simulink model "SVPWMv1"  (R2013a)
settings: Solver=ode45  StartTime=0.0  StopTime=2  MaxStep=.0001  RelTol=1e-3
libraries: powerlib x15, simulink x3, powerlib_meascontrol x1
settings Model: Creator=TELE  LastModifiedBy=TELE

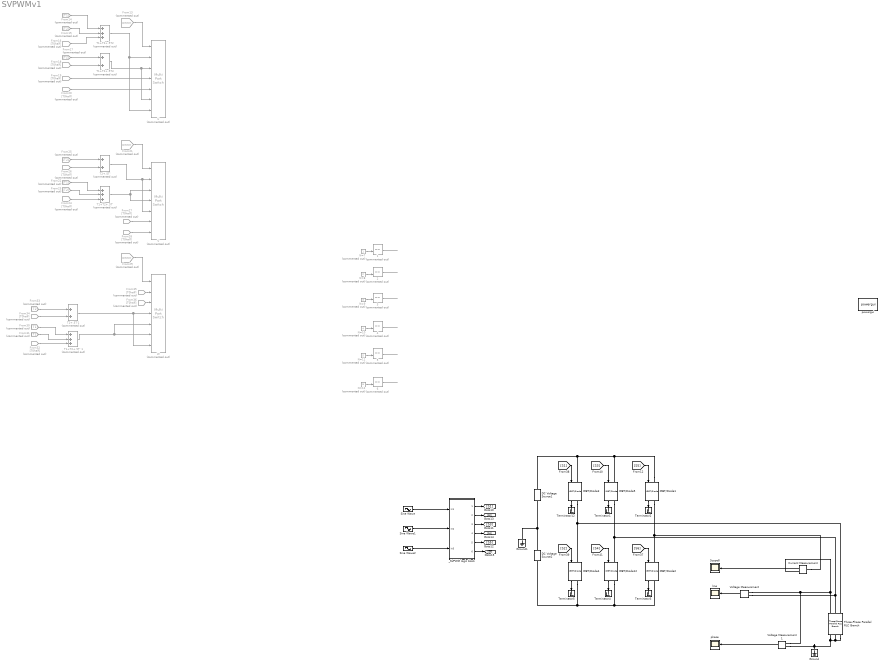
== system SVPWMv1 ==
  {1..6} (6 alike) : RelationalOperator  Commented=on  Operator===  OutDataTypeStr=boolean
  Current Measurement : powerlib/Measurements/Current Measurement  PhasorSimulation=off  OutputType=Complex  PSBequivalent=0
  DC Voltage Source1 : powerlib/Electrical Sources/DC Voltage Source  Amplitude=150  Measurements=None
  DC Voltage Source2 : powerlib/Electrical Sources/DC Voltage Source  Amplitude=150  Measurements=None
  From13 : From  Commented=on  GotoTag=sector
  From14 : From  Commented=on  GotoTag=T1
  From{15,17,23,25,31,33} (6 alike) : From  Commented=on  GotoTag=T2
  From{16,18..20,24,26..28,32,34..36} (12 alike) : From  Commented=on  GotoTag=T0half
  From21 : From  Commented=on  GotoTag=sector
  From22 : From  Commented=on  GotoTag=T1
  From29 : From  Commented=on  GotoTag=sector
  From30 : From  Commented=on  GotoTag=T1
  Ground : powerlib/Elements/Ground  LConnTagsString=a
  Ground1 : powerlib/Elements/Ground  LConnTagsString=a
  IGBT/Diode{1..5,12} (6 alike) : powerlib/Power Electronics/IGBT//Diode  Ron=1e-3  Rs=1e5  Cs=inf  Measurements=on
  N=10 : Constant  Commented=on  Value=4
  N=11 : Constant  Commented=on  Value=5
  N=12 : Constant  Commented=on  Value=6
  N=7 : Constant  Commented=on
  N=8 : Constant  Commented=on  Value=2
  N=9 : Constant  Commented=on  Value=3
  Scope8 : Scope
      settings: YMin=-600000  YMax=350000  SaveName=current
  Sine Wave : Sin  Frequency=50*2*pi  SampleTime=0
  Sine Wave1 : Sin  Frequency=50*2*pi  Phase=pi*(-2/3)  SampleTime=0
  Sine Wave2 : Sin  Frequency=50*2*pi  Phase=pi*(2/3)  SampleTime=0
  "T1+T2+.5T' " : Sum  Commented=on  Inputs=+++
  T1+T2+.5T' 1 : Sum  Commented=on  Inputs=+++
  T1+T2+.5T2 : Sum  Commented=on  Inputs=+++
  T1+T2+.5T3 : Sum  Commented=on  Inputs=2
  T2+.5T' : Sum  Commented=on  Inputs=2
  T2+.5T'1 : Sum  Commented=on  Inputs=2
  Terminator{1..5,12} (6 alike) : Terminator
  Three-Phase Parallel RLC Branch : powerlib/Elements/Three-Phase Parallel RLC Branch  LConnTagsString=A|B|C  RConnTagsString=A|B|C  BranchType=RLC  Resistance=100  Inductance=100e-3  Capacitance=100e-3  Measurements=None
  U : MultiPortSwitch  Commented=on  DataPortOrder=Specify indices  Inputs=4  DataPortIndices={1,2,3,4,5,6}
  V : MultiPortSwitch  Commented=on  DataPortOrder=Specify indices  Inputs=4  DataPortIndices={1,2,3,4,5,6}
  Voltage Measurement : powerlib/Measurements/Voltage Measurement  PhasorSimulation=off  OutputType=Complex  PSBequivalent=0
  Voltage Measurement1 : powerlib/Measurements/Voltage Measurement  PhasorSimulation=off  OutputType=Complex  PSBequivalent=0
  W : MultiPortSwitch  Commented=on  DataPortOrder=Specify indices  Inputs=4  DataPortIndices={1,2,3,4,5,6}
  _SVPWM logic block : Subsystem
  line : Scope
      settings: TimeRange=2  YMin=-175  YMax=175  SaveName=voltage
  phase : Scope
      settings: YMin=-10  YMax=150  SaveName=voltage1
  powergui : powerlib/powergui  Priority=1  SimulationMode=Continuous  SolverType=Tustin  SampleTime=50e-6  frequency=60  SPID=off  DisableSnubberDevices=off  DisableRonSwitches=off  DisableVfSwitches=off  SwTol=0  Interpol=off  DisplayEquations=off  frequencyindice=0  Pbase=100e6  ErrMax=1e-4  Iterations=50  UnitsV=kV  UnitsW=MW  FunctionMessages=off  echomessages=off  HookPort=off  EnableUseOfTLC=off  x0status=blocks  RestoreLinks=warning  ResistiveCurrentMeasurement=off  Frange=[0:2:500]  Ylog=off  Xlog=on  ShowGrid=off  save=off  variable=ZData  structure=voltage  ZoomFFT=off  StartTime=0.0  cycles=50  DisplayStyle=1  fundamental=50  FreqAxis=off  MaxFrequency=1000  frequencyindicesteady=1  RmsSteady=1  display=off  Ts=0  methode=off
  wires:
  ? -> 6/1, 5/1, 4/1, 3/1, 2/1, 1/1
  N=7/1 -> 1/2
  N=8/1 -> 2/2
  N=9/1 -> 3/2
  N=10/1 -> 4/2
  N=11/1 -> 5/2
  N=12/1 -> 6/2
  1/1 -> ?
  2/1 -> ?
  3/1 -> ?
  4/1 -> ?
  5/1 -> ?
  6/1 -> ?
  From13/1 -> U/1
  T1+T2+.5T2/1 -> U/2, U/7
  From14/1 -> T1+T2+.5T2/1
  From15/1 -> T1+T2+.5T2/2
  From16/1 -> T1+T2+.5T2/3
  From17/1 -> T1+T2+.5T3/1
  From18/1 -> T1+T2+.5T3/2
  T1+T2+.5T3/1 -> U/3, U/6
  From19/1 -> U/4
  From20/1 -> U/5
  From21/1 -> V/1
  From22/1 -> "T1+T2+.5T' "/1
  From23/1 -> "T1+T2+.5T' "/2
  From24/1 -> "T1+T2+.5T' "/3
  From25/1 -> T2+.5T'/1
  From26/1 -> T2+.5T'/2
  "T1+T2+.5T' "/1 -> V/4, V/3
  T2+.5T'/1 -> V/5, V/2
  From27/1 -> V/6
  From28/1 -> V/7
  From29/1 -> W/1
  From30/1 -> T1+T2+.5T' 1/1
  From31/1 -> T1+T2+.5T' 1/2
  From32/1 -> T1+T2+.5T' 1/3
  From33/1 -> T2+.5T'1/1
  From34/1 -> T2+.5T'1/2
  From35/1 -> W/2
  From36/1 -> W/3
  T2+.5T'1/1 -> W/7, W/4
  T1+T2+.5T' 1/1 -> W/6, W/5
  Voltage Measurement/1 -> line/1
  Current Measurement/1 -> Scope8/1
  Voltage Measurement1/1 -> phase/1
  _SVPWM logic block/6(6) -> [S6]
  [S6] -> IGBT/Diode2/1
  IGBT/Diode1/1 -> Terminator2/1
  _SVPWM logic block/2(2) -> [S2]
  IGBT/Diode4/1 -> Terminator5/1
  [S1] -> IGBT/Diode3/1
  IGBT/Diode5/1 -> Terminator1/1
  Sine Wave/1 -> _SVPWM logic block/1(In1)
  _SVPWM logic block/4(4) -> [S4]
  _SVPWM logic block/1(1) -> [S1]
  IGBT/Diode3/1 -> Terminator12/1
  IGBT/Diode2/1 -> Terminator3/1
  Sine Wave2/1 -> _SVPWM logic block/3(In3)
  [S3] -> IGBT/Diode5/1
  _SVPWM logic block/3(3) -> [S3]
  [S2] -> IGBT/Diode4/1
  [S5] -> IGBT/Diode1/1
  IGBT/Diode12/1 -> Terminator4/1
  [S4] -> IGBT/Diode12/1
  _SVPWM logic block/5(5) -> [S5]
  Sine Wave1/1 -> _SVPWM logic block/2(In2)
  connections:
  Voltage Measurement1/LConn2 -- Ground/LConn1 -- Three-Phase Parallel RLC Branch/LConn1 -- Three-Phase Parallel RLC Branch/LConn3 -- Three-Phase Parallel RLC Branch/LConn2
  DC Voltage Source1/LConn1 -- Ground1/LConn1 -- DC Voltage Source2/RConn1
  IGBT/Diode1/LConn1 -- DC Voltage Source1/RConn1 -- IGBT/Diode3/LConn1 -- IGBT/Diode5/LConn1
  IGBT/Diode2/RConn1 -- IGBT/Diode12/RConn1 -- DC Voltage Source2/LConn1 -- IGBT/Diode4/RConn1
  Voltage Measurement/LConn1 -- Current Measurement/RConn1 -- Three-Phase Parallel RLC Branch/RConn1 -- Voltage Measurement1/LConn1
  Voltage Measurement/LConn2 -- IGBT/Diode12/LConn1 -- IGBT/Diode5/RConn1 -- Three-Phase Parallel RLC Branch/RConn2
  IGBT/Diode3/RConn1 -- Three-Phase Parallel RLC Branch/RConn3 -- IGBT/Diode4/LConn1
  IGBT/Diode1/RConn1 -- Current Measurement/LConn1 -- IGBT/Diode2/LConn1

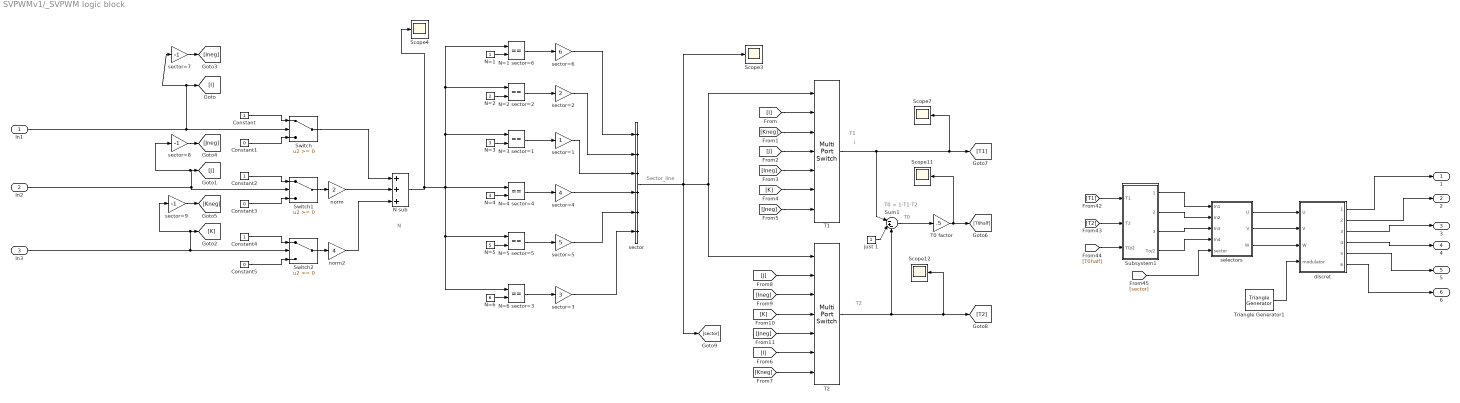
== system SVPWMv1/_SVPWM logic block ==
  note: T0
  note: T0 = 1-T1-T2
  note: T2
  note: T1
  note: i
  note: Sector_line
  note: N
  In1 : Inport
  In2 : Inport  Port=2
  In3 : Inport  Port=3
  Constant : Constant
  Constant1 : Constant  Value=0
  Constant2 : Constant
  Constant3 : Constant  Value=0
  Constant4 : Constant
  Constant5 : Constant  Value=0
  N sub : Sum  Inputs=+++
  N=1 : Constant
  N=1 sector=6 : RelationalOperator  Operator===  OutDataTypeStr=boolean
  N=2 : Constant  Value=2
  N=2 sector=2 : RelationalOperator  Operator===  OutDataTypeStr=boolean
  N=3 : Constant  Value=3
  N=3 sector=1 : RelationalOperator  Operator===  OutDataTypeStr=boolean
  N=4 : Constant  Value=4
  N=4 sector=4 : RelationalOperator  Operator===  OutDataTypeStr=boolean
  N=5 : Constant  Value=5
  N=5 sector=5 : RelationalOperator  Operator===  OutDataTypeStr=boolean
  N=6 : Constant  Value=6
  N=6 sector=3 : RelationalOperator  Operator===  OutDataTypeStr=boolean
  Scope{3..4,7,11..12} (5 alike) : Scope
      Scope11 settings: YMin=2.77556e-17  YMax=0.9  SaveName=current2
      Scope12 settings: YMin=2.77556e-17  YMax=0.9  SaveName=current3
      Scope3 settings: SaveName=ScopeData3
      Scope4 settings: SaveName=ScopeData4
      Scope7 settings: YMin=2.77556e-17  YMax=0.9  SaveName=current1
  Subsystem1 : Subsystem
  Sum1 : Sum  Inputs=|-+-
  Switch : Switch
  Switch1 : Switch
  Switch2 : Switch
  T0 factor : Gain  Gain=.5
  T1 : MultiPortSwitch  DataPortOrder=Specify indices  Inputs=4  DataPortIndices={1,2,3,4,5,6}
  T2 : MultiPortSwitch  DataPortOrder=Specify indices  Inputs=4  DataPortIndices={1,2,3,4,5,6}
  Triangle Generator1 : powerlib_meascontrol/Pulse & Signal Generators/Triangle Generator  Freq=50e3  Phase=180  Ts=0
  discret : Subsystem
  just 1 : Constant
  norm : Gain  Gain=2
  norm2 : Gain  Gain=4
  sector : Sum  Inputs=++++++
  sector=1 : Gain
  sector=2 : Gain  Gain=2
  sector=3 : Gain  Gain=3
  sector=4 : Gain  Gain=4
  sector=5 : Gain  Gain=5
  sector=6 : Gain  Gain=6
  sector=7 : Gain  Gain=-1
  sector=8 : Gain  Gain=-1
  sector=9 : Gain  Gain=-1
  selectors : Subsystem
  1 : Outport
  2 : Outport  Port=2
  3 : Outport  Port=3
  4 : Outport  Port=4
  5 : Outport  Port=5
  6 : Outport  Port=6
  wires:
  Constant1/1 -> Switch/3
  In1/1 -> Switch/2, sector=7/1, [I]
  Constant2/1 -> Switch1/1
  Constant/1 -> Switch/1
  Constant3/1 -> Switch1/3
  N=1/1 -> N=1 sector=6/2
  N=6/1 -> N=6 sector=3/2
  N=6 sector=3/1 -> sector=3/1
  N=5/1 -> N=5 sector=5/2
  N sub/1 -> Scope4/1, N=6 sector=3/1, N=5 sector=5/1, N=4 sector=4/1, N=3 sector=1/1, N=2 sector=2/1, N=1 sector=6/1
  N=3 sector=1/1 -> sector=1/1
  N=3/1 -> N=3 sector=1/2
  Constant4/1 -> Switch2/1
  Switch/1 -> N sub/1
  In2/1 -> Switch1/2, [J], sector=8/1
  N=4/1 -> N=4 sector=4/2
  N=5 sector=5/1 -> sector=5/1
  Switch2/1 -> norm2/1
  N=2/1 -> N=2 sector=2/2
  sector=2/1 -> sector/2
  N=2 sector=2/1 -> sector=2/1
  sector=4/1 -> sector/4
  sector=5/1 -> sector/5
  N=4 sector=4/1 -> sector=4/1
  sector=1/1 -> sector/3
  Switch1/1 -> norm/1
  sector=3/1 -> sector/6
  N=1 sector=6/1 -> sector=6/1
  sector=6/1 -> sector/1
  In3/1 -> Switch2/2, sector=9/1, [K]
  Constant5/1 -> Switch2/3
  [I] -> T1/2
  [Kneg] -> T2/7
  sector=8/1 -> [Jneg]
  Sum1/1 -> T0 factor/1
  T0 factor/1 -> Scope11/1, [T0half]
  sector/1 -> [sector], Scope3/1, T2/1, T1/1
  [Ineg] -> T1/5
  sector=7/1 -> [Ineg]
  norm2/1 -> N sub/3
  [Jneg] -> T1/7
  [J] -> T2/2
  [K] -> T1/6
  [J] -> T1/4
  [I] -> T2/6
  [K] -> T2/4
  T1/1 -> Scope7/1, [T1], Sum1/1
  sector=9/1 -> [Kneg]
  just 1/1 -> Sum1/2
  [Kneg] -> T1/3
  [Jneg] -> T2/5
  norm/1 -> N sub/2
  [Ineg] -> T2/3
  selectors/3(W) -> discret/3(W)
  Triangle Generator1/1 -> discret/4(modulator)
  discret/2(2) -> 2/1
  discret/3(3) -> 3/1
  Subsystem1/2(T1+To/2) -> selectors/2(In2)
  discret/4(4) -> 4/1
  Subsystem1/1(T1+T2+To/2) -> selectors/1(In1)
  [T1] -> Subsystem1/1(T1)
  [T0half] -> Subsystem1/3(T0/2)
  discret/1(1) -> 1/1
  T2/1 -> Sum1/3, Scope12/1, [T2]
  [T2] -> Subsystem1/2(T2)
  selectors/2(V) -> discret/2(V)
  Subsystem1/4(To/2) -> selectors/4(In4)
  [sector] -> selectors/5("sector ")
  Subsystem1/3(T2+To/2) -> selectors/3(In3)
  selectors/1(U) -> discret/1(U)
  discret/5(5) -> 5/1
  discret/6(6) -> 6/1

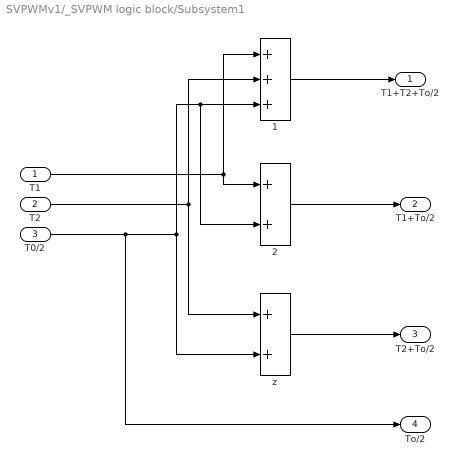
== system SVPWMv1/_SVPWM logic block/Subsystem1 ==
  T1 : Inport
  T2 : Inport  Port=2
  T0/2 : Inport  Port=3
  1 : Sum  Inputs=+++
  2 : Sum
  z : Sum
  T1+T2+To/2 : Outport
  T1+To/2 : Outport  Port=2
  T2+To/2 : Outport  Port=3
  To/2 : Outport  Port=4
  wires:
  T1/1 -> 2/1, 1/1
  T0/2/1 -> z/2, 1/3, 2/2, To/2/1
  2/1 -> T1+To/2/1
  1/1 -> T1+T2+To/2/1
  T2/1 -> z/1, 1/2
  z/1 -> T2+To/2/1

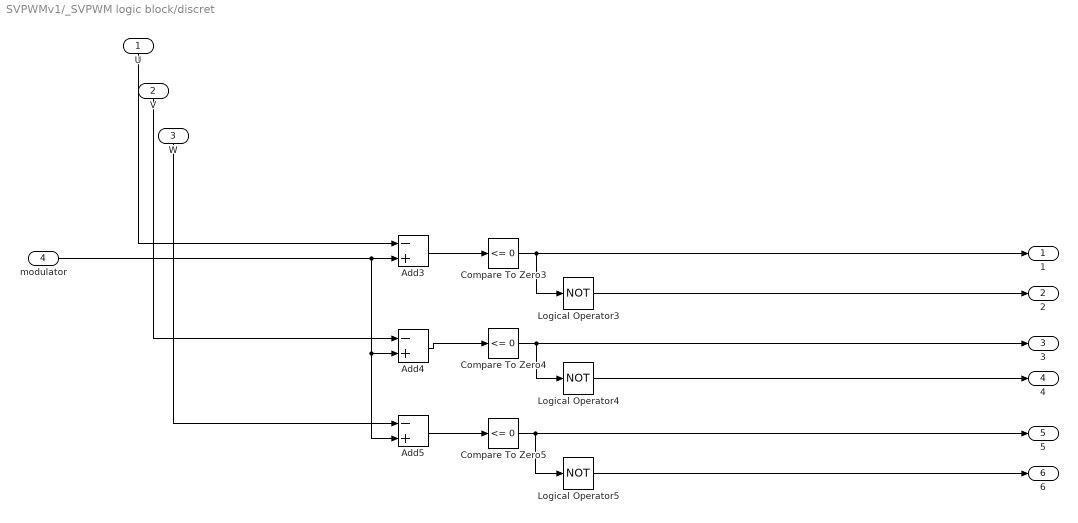
== system SVPWMv1/_SVPWM logic block/discret ==
  U : Inport
  V : Inport  Port=2
  W : Inport  Port=3
  modulator : Inport  Port=4
  Add3 : Sum  Inputs=-+
  Add4 : Sum  Inputs=-+
  Add5 : Sum  Inputs=-+
  Compare To Zero3 : simulink/Logic and Bit Operations/Compare To Zero  relop=<=  OutDataTypeStr=boolean
  Compare To Zero4 : simulink/Logic and Bit Operations/Compare To Zero  relop=<=  OutDataTypeStr=boolean
  Compare To Zero5 : simulink/Logic and Bit Operations/Compare To Zero  relop=<=  OutDataTypeStr=boolean
  Logical Operator3 : Logic  Operator=NOT  AllPortsSameDT=off  OutDataTypeStr=boolean
  Logical Operator4 : Logic  Operator=NOT  AllPortsSameDT=off  OutDataTypeStr=boolean
  Logical Operator5 : Logic  Operator=NOT  AllPortsSameDT=off  OutDataTypeStr=boolean
  1 : Outport
  2 : Outport  Port=2
  3 : Outport  Port=3
  4 : Outport  Port=4
  5 : Outport  Port=5
  6 : Outport  Port=6
  wires:
  Compare To Zero4/1 -> Logical Operator4/1, 3/1
  Compare To Zero5/1 -> Logical Operator5/1, 5/1
  Logical Operator3/1 -> 2/1
  Compare To Zero3/1 -> Logical Operator3/1, 1/1
  Logical Operator4/1 -> 4/1
  Logical Operator5/1 -> 6/1
  V/1 -> Add4/1
  W/1 -> Add5/1
  U/1 -> Add3/1
  Add5/1 -> Compare To Zero5/1
  Add3/1 -> Compare To Zero3/1
  Add4/1 -> Compare To Zero4/1
  modulator/1 -> Add3/2, Add5/2, Add4/2

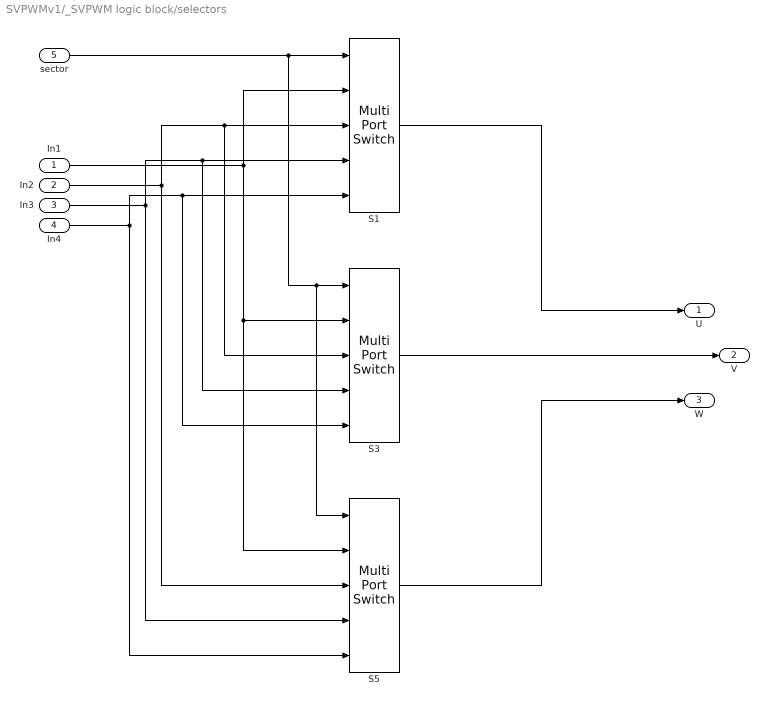
== system SVPWMv1/_SVPWM logic block/selectors ==
  In1 : Inport
  In2 : Inport  Port=2
  In3 : Inport  Port=3
  In4 : Inport  Port=4
  "sector " : Inport  Port=5
  S1 : MultiPortSwitch  DataPortOrder=Specify indices  Inputs=4  DataPortIndices={[1,6],2,5,[3,4]}
  S3 : MultiPortSwitch  DataPortOrder=Specify indices  Inputs=4  DataPortIndices={[2,3],4,1,[5,6]}
  S5 : MultiPortSwitch  DataPortOrder=Specify indices  Inputs=4  DataPortIndices={[4,5],6,3,[1,2]}
  U : Outport
  V : Outport  Port=2
  W : Outport  Port=3
  wires:
  S1/1 -> U/1
  In4/1 -> S5/5, S1/5, S3/5
  In1/1 -> S3/2, S5/2, S1/2
  In2/1 -> S5/3, S1/3, S3/3
  S5/1 -> W/1
  In3/1 -> S5/4, S1/4, S3/4
  S3/1 -> V/1
  "sector "/1 -> S5/1, S3/1, S1/1
